simulink model "bit_mapping_model"  (R2020b)
settings: Solver=FixedStepDiscrete  StartTime=0.0  StopTime=10.0  RelTol=1e-3
libraries: commrandsrc3 x1, hdlsllib x1
settings Model: DataTypeOverride=Off  Creator=wardo  LastModifiedBy=EFlores
settings OptimizationCC: BlockReduction=off  ConditionallyExecuteInputs=off  DefaultParameterBehavior=Inlined
settings DebuggingCC: AlgebraicLoopMsg=error  SingleTaskRateTransMsg=error
settings HardwareCC: ProdBitPerPointer=32  ProdBitPerSizeT=32  ProdBitPerPtrDiffT=32  ProdLargestAtomicFloat=None  ProdIntDivRoundTo=Undefined  ProdEndianess=Unspecified  ProdWordSize=32  ProdHWDeviceType=ASIC/FPGA->ASIC/FPGA  TargetBitPerPointer=64  TargetBitPerSizeT=64  TargetBitPerPtrDiffT=64  TargetLongLongMode=on  TargetIntDivRoundTo=Zero  TargetEndianess=LittleEndian  TargetWordSize=64  TargetHWDeviceType=Custom Processor->MATLAB Host Computer  ProdEqTarget=off

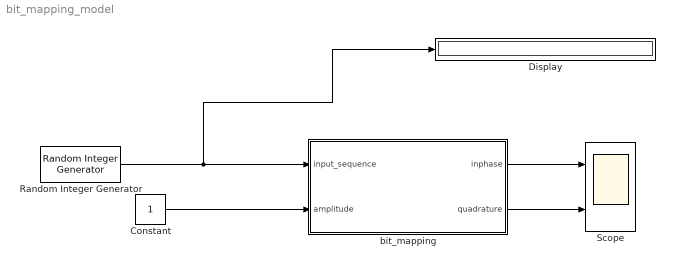
== system bit_mapping_model ==
  Constant : Constant  OutMin=0  OutMax=5  OutDataTypeStr=fixdt(1,16)  SampleTime=-1
  Display : Display
  Random Integer Generator : commrandsrc3/Random Integer Generator  SetSize=2  SeedSource=Auto  Seed=0  SampleTime=1  SamplesPerFrame=3  OutputDataType=boolean  SimulateUsing=Interpreted execution
  Scope : Scope  NumInputPorts=2
  bit_mapping : Subsystem
  wires:
  bit_mapping/2(quadrature) -> Scope/2
  Constant/1 -> bit_mapping/2(amplitude)
  Random Integer Generator/1 -> Display/1, bit_mapping/1(input_sequence)
  bit_mapping/1(inphase) -> Scope/1

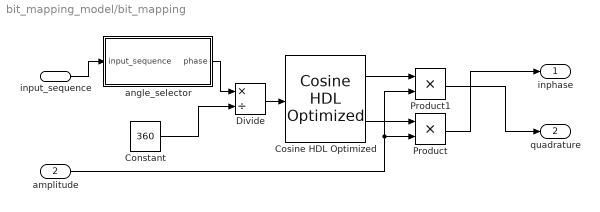
== system bit_mapping_model/bit_mapping ==
  input_sequence : Inport
  amplitude : Inport  Port=2
  Constant : Constant  Value=360  OutDataTypeStr=fixdt(0,9,0)  SampleTime=-1
  Cosine HDL Optimized : hdlsllib/Lookup Tables/Cosine HDL Optimized  OutputFormula=sin(2*pi*u) and cos(2*pi*u)  NumDataPoints=64  TableDataTypeStr=fixdt(1,16,15)  SimulateLUTROMDelay=off
      settings: SourceProductBaseCode=SL
  Divide : Product  Inputs=*/  OutMin=0  OutMax=1  OutDataTypeStr=fixdt(1,16,14)  RndMeth=Zero  SaturateOnIntegerOverflow=on
  Product : Product
  Product1 : Product
  angle_selector : MATLAB Function  TreatAsAtomicUnit=on
  inphase : Outport  VectorParamsAs1DForOutWhenUnconnected=off
  quadrature : Outport  Port=2  VectorParamsAs1DForOutWhenUnconnected=off
  wires:
  Product/1 -> inphase/1
  Product1/1 -> quadrature/1
  input_sequence/1 -> angle_selector/1(input_sequence)
  amplitude/1 -> Product1/2, Product/2
  Cosine HDL Optimized/2 -> Product/1
  Cosine HDL Optimized/1 -> Product1/1
  Divide/1 -> Cosine HDL Optimized/1
  angle_selector/1(phase) -> Divide/1
  Constant/1 -> Divide/2

== matlab function bit_mapping_model/bit_mapping/angle_selector ==
  settings: fimath=fimath('RoundingMethod', 'Floor','OverflowAction', 'Wrap','ProductMode', 'FullPrecision', 'SumMode', 'FullPrecision')
  data: input_sequence input; phase output
function phase = phase_selector(input_sequence)
%#codegen
% Receives a bit sequence and returns the angle in radians of the
% corresponding 8-psk constellation symbol. Gray encoding is used as stated
% in the DVB-S2 standard.
    tmp = 0; % Start at phase 0
    if(input_sequence(1)==0 && input_sequence(2)==0 && input_sequence(3)==1)
        tmp=0;
    elseif(input_sequence(1)==0 && input_sequence(2)==0 && input_sequence(3)==0)
        tmp=45;
    elseif(input_sequence(1)==1 && input_sequence(2)==0 && input_sequence(3)==0)
        tmp=90;
    elseif(input_sequence(1)==1 && input_sequence(2)==1 && input_sequence(3)==0)
        tmp=135;
    elseif(input_sequence(1)==0 && input_sequence(2)==1 && input_sequence(3)==0)
        tmp=180;
    elseif(input_sequence(1)==0 && input_sequence(2)==1 && input_sequence(3)==1)
        tmp=225;
    elseif(input_sequence(1)==1 && input_sequence(2)==1 && input_sequence(3)==1)
        tmp=270;
    elseif(input_sequence(1)==1 && input_sequence(2)==0 && input_sequence(3)==1)
        tmp=315;
    end
    % 9 bits necessary to represent 360 degrees.
    phase = fi(tmp, 0, 23, 14, hdlfimath);
